simulink model "sim_final_VSS_PWM"  (R2019a)
settings: Solver=ode8  StartTime=0.0  StopTime=end_time  FixedStep=FStep  RelTol=1e-3  EnableMultiTasking=on
undefined symbols (not defined in the file): a, b, C1, C2, d, ds, h, K, k1, k2, T, x0, y0, z0, zad
libraries: simulink x2, simulink_extras x1
settings Model: Creator=user  LastModifiedBy=ogure
settings SolverCC: SolverResetMethod=Robust
settings DataIOCC: LimitDataPoints=on  SaveFormat=Array  SaveOutput=off  ReturnWorkspaceOutputs=off  OutputSaveName=X,X1,X2,X3,X4,L,H
settings OptimizationCC: LifeSpan=inf
settings DebuggingCC: SolverPrmCheckMsg=warning  MultiTaskRateTransMsg=warning  SFUnexpectedBacktrackingDiag=warning  SFNoUnconditionalDefaultTransitionDiag=warning  SFExecutionAtInitializationDiag=none  ArithmeticOperatorsInVariantConditions=warning
settings HardwareCC: ProdBitPerPointer=32  ProdBitPerSizeT=32  ProdBitPerPtrDiffT=32  ProdLargestAtomicFloat=None  ProdIntDivRoundTo=Undefined  ProdEndianess=Unspecified  ProdWordSize=32  ProdHWDeviceType=32-bit Generic
settings ModelReferenceCC: PropagateSignalLabelsOutOfModel=off
settings SFSimCC: SimUseLocalCustomCode=off
settings RTWCC: RTWUseLocalCustomCode=off
settings CodeAppCC: StateflowObjectComments=on
settings GRTTargetCC: TargetLangStandard=C89/C90 (ANSI)  GeneratePreprocessorConditionals=Disable all
settings ConfigComp: CovMetricSettings=dw  CovHtmlReporting=on  CovSaveCumulativeToWorkspaceVar=on  CovSaveSingleToWorkspaceVar=on  CovExternalEMLEnable=off  CovSFcnEnable=off

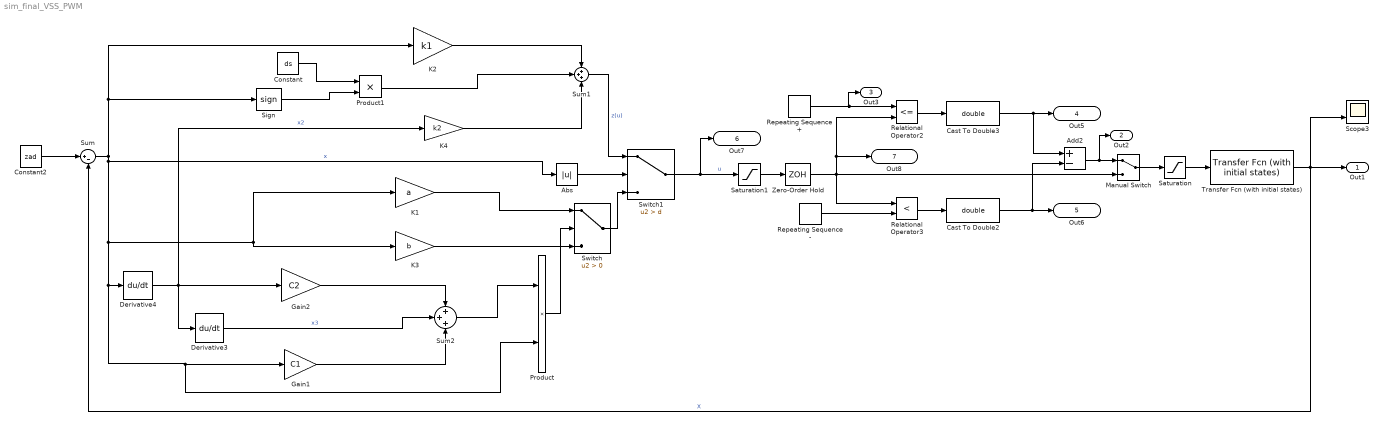
== system sim_final_VSS_PWM ==
  Abs : Abs
  Add2 : Sum  Inputs=+-
  Cast To Double2 : DataTypeConversion  OutDataTypeStr=double
  Cast To Double3 : DataTypeConversion  OutDataTypeStr=double
  Constant : Constant  Value=ds
  Constant2 : Constant  Value=zad
  Derivative3 : Derivative  CoefficientInTFapproximation=0.00000001
  Derivative4 : Derivative  CoefficientInTFapproximation=0.00000001
  Gain1 : Gain  Gain=C1
  Gain2 : Gain  Gain=C2
  K1 : Gain  Gain=a
  K2 : Gain  Gain=k1
  K3 : Gain  Gain=b
  K4 : Gain  Gain=k2
  Manual Switch : ManualSwitch
  Product : Product
  Product1 : Product
  Relational Operator2 : RelationalOperator  Operator=<=  OutDataTypeStr=boolean  ZeroCross=off  RndMeth=Simplest
  Relational Operator3 : RelationalOperator  Operator=<  OutDataTypeStr=boolean  ZeroCross=off  RndMeth=Simplest
  Repeating Sequence + : simulink/Sources/Repeating Sequence  rep_seq_t=[0 0.1]  rep_seq_y=[0 d]
  Repeating Sequence - : simulink/Sources/Repeating Sequence  rep_seq_t=[0 0.1]  rep_seq_y=[0 d]
  Saturation : Saturate  UpperLimit=d  LowerLimit=-d
  Saturation1 : Saturate  UpperLimit=d  LowerLimit=-d
  Scope3 : Scope  NumInputPorts=2
  Sign : Signum
  Sum : Sum  Inputs=|+-
  Sum1 : Sum  Inputs=+++
  Sum2 : Sum  Inputs=+++
  Switch : Switch  Criteria=u2 > Threshold  ZeroCross=off
  Switch1 : Switch  Criteria=u2 > Threshold  Threshold=d  ZeroCross=off
  Transfer Fcn (with initial states) : simulink_extras/Additional Linear/Transfer Fcn (with initial states)  N=K  D=[T^2 2*h*T 1 0]  X0=[z0 y0 x0]
  Zero-Order Hold : ZeroOrderHold  SampleTime=0.1
  Out1 : Outport  SignalName=X
  Out2 : Outport  Port=2  SignalName=PWm
  Out3 : Outport  Port=3  SignalName=saw
  Out5 : Outport  Port=4  SignalName=pwm1
  Out6 : Outport  Port=5  SignalName=pwm2
  Out7 : Outport  Port=6  SignalName=upr
  Out8 : Outport  Port=7  SignalName=upr_ogr
  wires:
  Transfer Fcn (with initial states)/1 -> Scope3/2, Sum/2, Out1/1  "X"
  Derivative3/1 -> Sum2/2  "x3"
  Gain1/1 -> Sum2/3
  Sum2/1 -> Product/1
  K1/1 -> Switch/1
  Sum/1 -> Abs/1, K1/1, K3/1, Gain1/1, Product/2, Derivative4/1, K2/1, Sign/1  "x"
  Derivative4/1 -> K4/1, Gain2/1, Derivative3/1  "x2"
  Product/1 -> Switch/2
  Gain2/1 -> Sum2/1
  K3/1 -> Switch/3
  Switch/1 -> Switch1/3
  Sign/1 -> Product1/2
  Constant/1 -> Product1/1
  K2/1 -> Sum1/1
  K4/1 -> Sum1/3
  Product1/1 -> Sum1/2
  Constant2/1 -> Sum/1
  Sum1/1 -> Switch1/1  "z(u)"
  Abs/1 -> Switch1/2
  Switch1/1 -> Out7/1, Saturation1/1  "u"
  Saturation/1 -> Transfer Fcn (with initial states)/1
  Zero-Order Hold/1 -> Out8/1, Relational Operator2/2, Manual Switch/2, Relational Operator3/1
  Repeating Sequence +/1 -> Out3/1, Relational Operator2/1
  Cast To Double3/1 -> Out5/1, Add2/1
  Repeating Sequence -/1 -> Relational Operator3/2
  Cast To Double2/1 -> Out6/1, Add2/2
  Relational Operator3/1 -> Cast To Double2/1
  Relational Operator2/1 -> Cast To Double3/1
  Add2/1 -> Out2/1, Manual Switch/1
  Manual Switch/1 -> Saturation/1
  Saturation1/1 -> Zero-Order Hold/1
